simulink model "exp2_Real"  (R2018b)
settings: Solver=VariableStepAuto  StartTime=0.0  StopTime=10.0  RelTol=1e-3
libraries: simulink_extras x1
settings Model: Creator=LEGION  LastModifiedBy=LEGION

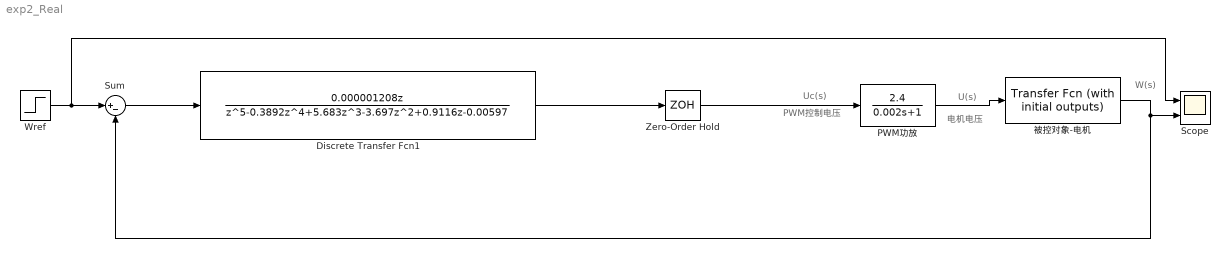
== system exp2_Real ==
  note: PWM控制电压
  note: Uc(s)
  note: 电机电压
  note: U(s)
  note: W(s)
  Discrete Transfer Fcn1 : DiscreteTransferFcn  Numerator=[0.000001208 0]  Denominator=[1 -0.3892 5.683 -3.697 0.9116 -0.00597]  SampleTime=0.01
  PWM功放 : TransferFcn  Numerator=[2.4 ]  Denominator=[0.002 1]
  Scope : Scope  NumInputPorts=2
  Sum : Sum  Inputs=|+-
  "Wref " : Step  Time=0  SampleTime=0
  Zero-Order Hold : ZeroOrderHold  SampleTime=0.01
  "被控对象-电机 " : simulink_extras/Additional Linear/Transfer Fcn (with initial outputs)  N=[0.01]  D=[0.005 0.06 0.1]  Y0=0  U0=0
  wires:
  "被控对象-电机 "/1 -> Sum/2, Scope/2
  PWM功放/1 -> "被控对象-电机 "/1
  "Wref "/1 -> Scope/1, Sum/1
  Sum/1 -> Discrete Transfer Fcn1/1
  Discrete Transfer Fcn1/1 -> Zero-Order Hold/1
  Zero-Order Hold/1 -> PWM功放/1
